simulink model "DECODER"  (R2016a)
settings: Solver=VariableStepAuto  StartTime=0.0  StopTime=0.5  RelTol=1e-3
undefined symbols (not defined in the file or in its folder): data
libraries: commcnvcod2 x2, commchan3 x1, commrandsrc3 x1, commsink2 x1
settings Model: Creator=Orza  LastModifiedBy=Orza

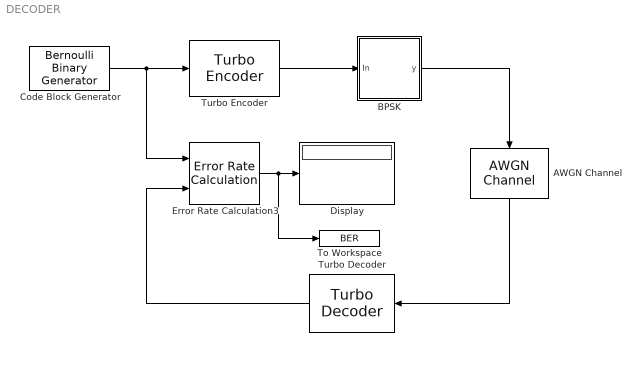
== system DECODER ==
  AWGN Channel : commchan3/AWGN Channel  InputProcessing=Columns as channels (frame based)  seed=67  noiseMode=Variance from mask  EbNodB=10  EsNodB=10  SNRdB=10  bitsPerSym=1  Ps=1  Tsym=1  variance=data.NoiseVar
  BPSK : Subsystem
      mask Display: disp(['BPSK']);
  Code Block Generator : commrandsrc3/Bernoulli Binary Generator  ProbabilityOfZero=0.5  SeedSource=Parameter  Seed=12345  SampleTime=1/data.BlockLength  SamplesPerFrame=data.BlockLength  OutputDataType=double  SimulateUsing=Interpreted execution
  Display : Display
  Error Rate Calculation3 : commsink2/Error Rate Calculation  N=0  st_delay=0  cp_mode=Entire frame  subframe=[]  PMode=Port  WsName=ErrorVec1  RsMode2=off  stop=off  numErr=maxNumErrs  maxBits=maxNumBits
  To Workspace : ToWorkspace  VariableName=BER  SampleTime=-1
      settings: MaxDataPoints=1
  Turbo Decoder : commcnvcod2/Turbo Decoder  TrellisStructure=data.trellis  InterleaverIndicesSource=Property  InterleaverIndices=data.InterleaverIndices  Algorithm=True APP  NumScalingBits=3  NumIterations=data.NoIter  SimulateUsing=Interpreted execution
  Turbo Encoder : commcnvcod2/Turbo Encoder  TrellisStructure=data.trellis  InterleaverIndicesSource=Property  InterleaverIndices=data.InterleaverIndices  SimulateUsing=Interpreted execution
  wires:
  Code Block Generator/1 -> Error Rate Calculation3/1, Turbo Encoder/1
  AWGN Channel/1 -> Turbo Decoder/1
  Turbo Decoder/1 -> Error Rate Calculation3/2
  Error Rate Calculation3/1 -> To Workspace/1, Display/1
  BPSK/1(y) -> AWGN Channel/1
  Turbo Encoder/1 -> BPSK/1(In)

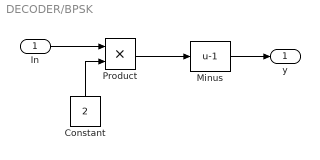
== system DECODER/BPSK ==
  In : Inport
  Constant : Constant  Value=2
  Minus : Bias  Bias=-1
  Product : Product
  y : Outport
  wires:
  In/1 -> Product/1
  Constant/1 -> Product/2
  Product/1 -> Minus/1
  Minus/1 -> y/1
